simulink subsystem "target"  (R2024b)
settings: Solver=VariableStepAuto  StartTime=0.0  StopTime=10.0  RelTol=1e-3
settings Model: Creator=yagiz  LastModifiedBy=yagiz

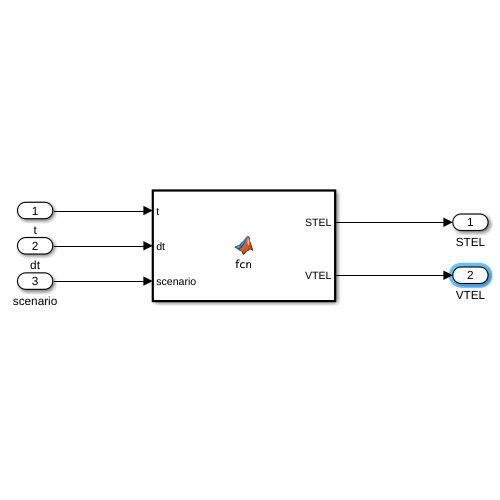
[thumbnail: Simulink's stored preview of the top-level diagram]
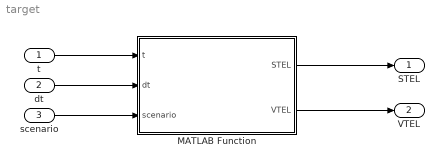
== system target ==
  t : Inport
  dt : Inport  Port=2
  scenario : Inport  Port=3
  MATLAB Function : MATLAB Function  TreatAsAtomicUnit=on
  STEL : Outport
  VTEL : Outport  Port=2
  wires:
  t/1 -> MATLAB Function/1(t)
  dt/1 -> MATLAB Function/2(dt)
  scenario/1 -> MATLAB Function/3(scenario)
  MATLAB Function/1(STEL) -> STEL/1
  MATLAB Function/2(VTEL) -> VTEL/1

== matlab function target/MATLAB Function ==
  settings: updateMethod=DISCRETE
  data: t input; STEL output; dt input; scenario input; VTEL output
function [STEL, VTEL] = fcn(t, dt, scenario)

persistent pos vel initialized

G = 9.80665;

% Initial conditions per scenario
IC = {
    [6000,  1500, -10000], [-200,  0,   0];   % S1
    [6000,  1500, -10000], [-200,  0,   0];   % S2
    [6000,  1500, -10000], [-200,  0,   0];   % S3
    [6000,  1500, -10000], [-200,  0,   0];   % S4
    [5500, -2000, -10000], [   0, 300,  0];   % S5
    [7000,     0, -10000], [-300,  0,   0];   % S6
    [5500,  1000,  -7500], [-220,  0,   0];   % S7
    [6000,  1500, -10000], [-200,  0,   0];   % S8
    [6500,   800, -10000], [-250,  0,   0];   % S9
    [10000,-1000, -12000], [-180, 120,  0];   % S10
};

if isempty(initialized)
    pos = IC{scenario,1}';
    vel = IC{scenario,2}';
    initialized = true;
end

% Compute acceleration
acc = target_accel(scenario, t, vel, G);

% S1: analytic (constant velocity)
if scenario == 1
    p0 = IC{scenario,1}';
    v0 = IC{scenario,2}';
    STEL = p0 + v0 * t;
    VTEL = v0;
    return;
end

% Euler integration for S2-S10
vel_new = vel + acc * dt;
pos_new = pos + vel * dt;

pos = pos_new;
vel = vel_new;

STEL = pos;
VTEL = vel;

function acc = target_accel(s, t, vel, G)
acc = zeros(3,1);

vn = vel(1); ve = vel(2);
mag = sqrt(vn^2 + ve^2);
if mag > 1.0
    cw = [ve/mag; -vn/mag; 0];
else
    cw = zeros(3,1);
end

if s == 2
    if t >= 1.5, acc = 5.0*G*cw; end

elseif s == 3
    acc = [0; 3.0*G*sin(1.2*t); -2.0*G*cos(1.8*t + pi/3)];

elseif s == 4
    if t < 2.0,     acc = zeros(3,1);
    elseif t < 3.5, acc = 8.0*G*cw;
    elseif t < 4.8, acc = [0; 0; -6.0*G];
    end

elseif s == 6
    if t >= 3.0 && t < 8.0, acc = 7.0*G*cw; end

elseif s == 8
    if t >= 4.0, acc = [0; 6.364*G; -6.364*G]; end

elseif s == 9
    vm = norm(vel);
    if vm > 1.0
        vhat = vel/vm;
        a_drag = -0.7*G*vhat;
        up = [0;0;-1];
        perp = up - dot(up,vhat)*vhat;
        pm = norm(perp);
        if pm > 1e-6
            a_lift = 3.0*G*perp/pm;
        else
            a_lift = zeros(3,1);
        end
        acc = a_drag + a_lift;
    end

elseif s == 10
    vm = sqrt(vel(1)^2 + vel(2)^2);
    if vm > 0.1
        acc = [-vel(2)/vm*4.0*G; vel(1)/vm*4.0*G; 0];
    end
end
